simulink model "Arritmia"  (R2023a)
settings: Solver=ode15s  StartTime=0  StopTime=5  MaxStep=1e-3  RelTol=1e-3
libraries: slpidlib x1
settings Model: Creator=piqui  LastModifiedBy=jaelb
settings DataIOCC: ReturnWorkspaceOutputs=off  TimeSaveName=t
settings DebuggingCC: AlgebraicLoopMsg=none  ArtificialAlgebraicLoopMsg=none  MaxConsecutiveZCsMsg=none  ModelReferenceExtraNoncontSigs=none  OperatingPointInterfaceChecksumMismatchMsg=none

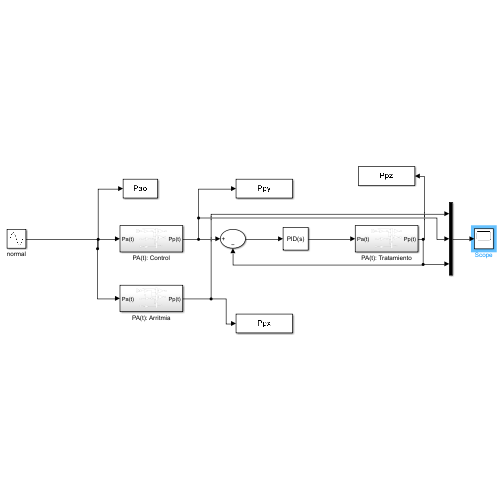
[thumbnail: Simulink's stored preview of the top-level diagram]
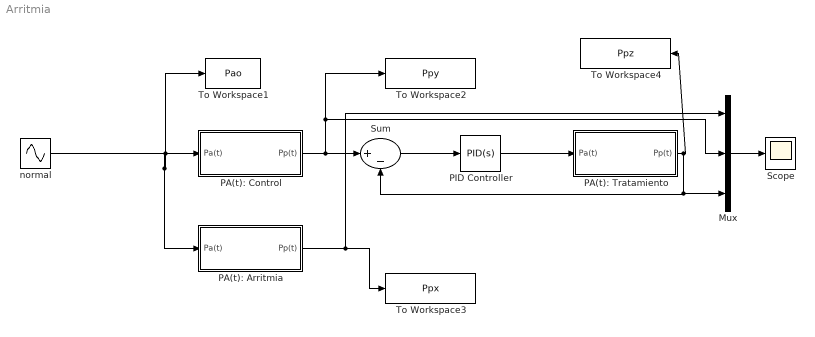
== system Arritmia ==
  Mux : Mux  Inputs=3
  PA(t): Arritmia : Subsystem
  PA(t): Control : Subsystem
  PA(t): Tratamiento : Subsystem
  PID Controller : slpidlib/PID Controller  Controller=PID  Form=Parallel  TimeDomain=Continuous-time  UseExternalTs=off  SampleTime=-1  IntegratorMethod=Forward Euler  FilterMethod=Forward Euler  ControllerParametersSource=internal  P=1382.64108107363  I=23976.1659464632  UseKiTs=off  D=7.06671657792426  N=251170.983745407  UseFilter=on  TunerSelectOption=Transfer Function Based (PID Tuner App)  InitialConditionSource=internal  InitialConditionForIntegrator=0  InitialConditionForFilter=0  DifferentiatorICPrevScaledInput=0  ExternalReset=none  TrackingMode=off  Kt=1  LimitOutput=off  SatLimitsSource=internal  UpperSaturationLimit=inf  LowerSaturationLimit=-inf  LinearizeAsGain=on  AntiWindupMode=none  Kb=1  LimitIntegrator=off  UpperIntegratorSaturationLimit=inf  LowerIntegratorSaturationLimit=-inf  POutMin=[]  POutMax=[]  IOutMin=[]  IOutMax=[]  DOutMin=[]  DOutMax=[]  NOutMin=[]  NOutMax=[]  SumOutMin=[]  SumOutMax=[]  SaturationOutMin=[]  SaturationOutMax=[]  PParamMin=[]  PParamMax=[]  IParamMin=[]  IParamMax=[]  DParamMin=[]  DParamMax=[]  NParamMin=[]  NParamMax=[]  KbParamMin=[]  KbParamMax=[]  KtParamMin=[]  KtParamMax=[]  KbOutMin=[]  KbOutMax=[]  KtOutMin=[]  KtOutMax=[]  IntegratorOutMin=[]  IntegratorOutMax=[]  FilterOutMin=[]  FilterOutMax=[]  SumI1OutMin=[]  SumI1OutMax=[]  SumI2OutMin=[]  SumI2OutMax=[]  SumI3OutMin=[]  SumI3OutMax=[]  SumI4OutMin=[]  SumI4OutMax=[]  SumDOutMin=[]  SumDOutMax=[]  DifferentiatorOutMin=[]  DifferentiatorOutMax=[]  FilterDiffOutCoefMin=[]  FilterDiffOutCoefMax=[]  ReciprocalOutMin=[]  ReciprocalOutMax=[]  SumDenOutMin=[]  SumDenOutMax=[]  SumNumOutMin=[]  SumNumOutMax=[]  DivideOutMin=[]  DivideOutMax=[]  UdiffTsProdOutMin=[]  UdiffTsProdOutMax=[]  NTsProdOutMin=[]  NTsProdOutMax=[]  UintegralTsProdOutMin=[]  UintegralTsProdOutMax=[]  UngainTsProdOutMin=[]  UngainTsProdOutMax=[]  ClampingZeroOutDataTypeStr=Inherit: Inherit via back propagation  ClampingZeroOutMin=[]  ClampingZeroOutMax=[]  FilterDenConstantOutDataTypeStr=Inherit: Inherit via back propagation  FilterDenConstantOutMin=[]  FilterDenConstantOutMax=[]  PCopyOutDataTypeStr=Inherit: Inherit via back propagation  PCopyOutMin=[]  PCopyOutMax=[]  NCopyOutDataTypeStr=Inherit: Inherit via back propagation  NCopyOutMin=[]  NCopyOutMax=[]  IntegratorContinuousStateAttributes=''  IntegratorStateMustResolveToSignalObject=off  IntegratorRTWStateStorageClass=Auto  FilterContinuousStateAttributes=''  FilterStateMustResolveToSignalObject=off  FilterRTWStateStorageClass=Auto  ParallelPVariant=InternalParameters  IdealPVariant=Disabled  IVariant=InternalParameters  DVariant=InternalParameters  IntegratorVariant=Continuous  SatVariant=Disabled  AWVariant=Passthrough  PCopyVariant=Disabled  TRVariant=Disabled  FdbkBlocksVariant=Forward  IdealPFdbkVariant=Disabled  SatFdbkVariant=Disabled  DerivativeFilterVariant=ContFilter  NVariant=InternalParameters  NCopyVariant=Disabled  FilterICVariant=InternalICsFilter  IntegratorICVariant=InternalICs  ExternalResetVariant=Disabled  TRSumVariant=Passthrough  SumFdbkVariant=Disabled  SumVariant=Sum_PID  TsampFilterVariant=InternalTs  TsampNgainVariant=Passthrough  TsampIntegralVariant=Disabled_SignalSpec  ExternalSaturationOutDataTypeStr=Inherit: Same as second input
  Scope : Scope
  Sum : Sum  Inputs=|+-
  To Workspace1 : ToWorkspace  VariableName=Pao  SampleTime=-1
  To Workspace2 : ToWorkspace  VariableName=Ppy  SampleTime=-1
  To Workspace3 : ToWorkspace  VariableName=Ppx  SampleTime=-1
  To Workspace4 : ToWorkspace  VariableName=Ppz  SampleTime=-1
  normal : Sin  Frequency=pi*2  SampleTime=0
  wires:
  normal/1 -> PA(t): Arritmia/1(Pa(t)), PA(t): Control/1(Pa(t)), To Workspace1/1
  Sum/1 -> PID Controller/1
  Mux/1 -> Scope/1
  PA(t): Control/1(Pp(t)) -> Mux/2, To Workspace2/1, Sum/1
  PA(t): Arritmia/1(Pp(t)) -> Mux/1, To Workspace3/1
  PID Controller/1 -> PA(t): Tratamiento/1(Pa(t))
  PA(t): Tratamiento/1(Pp(t)) -> Mux/3, Sum/2, To Workspace4/1

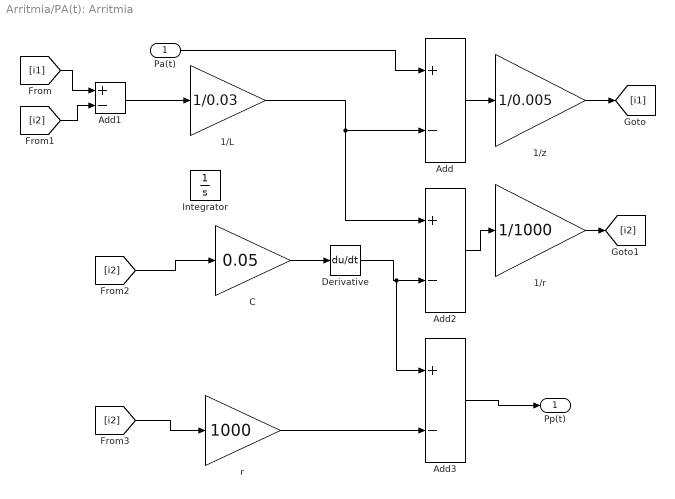
== system Arritmia/PA(t): Arritmia ==
  Pa(t) : Inport
  1/L : Gain  Gain=1/0.03
  1/r : Gain  Gain=1/1000
  1/z : Gain  Gain=1/0.005
  Add{,1..3} (4 alike) : Sum  Inputs=+-
  C : Gain  Gain=0.05
  Derivative : Derivative
  Integrator : Integrator
  r : Gain  Gain=1000
  Pp(t) : Outport
  wires:
  1/L/1 -> Add2/1, Add/2
  1/z/1 -> [i1]
  [i1] -> Add1/1
  Add2/1 -> 1/r/1
  Add3/1 -> Pp(t)/1
  r/1 -> Add3/2
  Pa(t)/1 -> Add/1
  Add/1 -> 1/z/1
  Derivative/1 -> Add3/1, Add2/2
  Add1/1 -> 1/L/1
  1/r/1 -> [i2]
  C/1 -> Derivative/1
  [i2] -> Add1/2
  [i2] -> C/1
  [i2] -> r/1

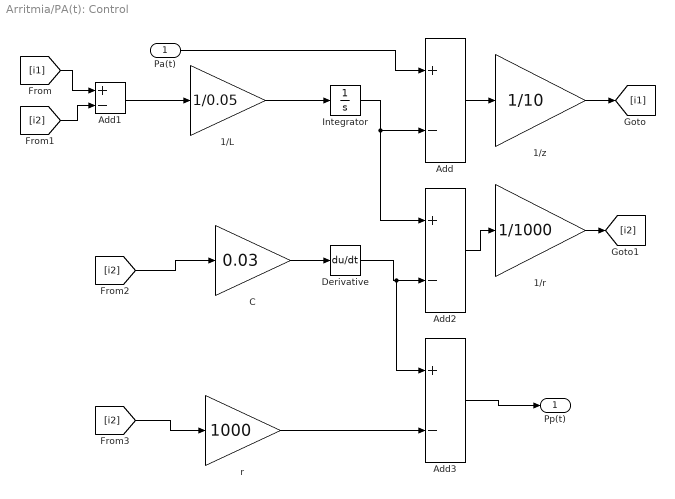
== system Arritmia/PA(t): Control ==
  Pa(t) : Inport
  1/L : Gain  Gain=1/0.05
  1/r : Gain  Gain=1/1000
  1/z : Gain  Gain=1/10
  Add{,1..3} (4 alike) : Sum  Inputs=+-
  C : Gain  Gain=0.03
  Derivative : Derivative
  Integrator : Integrator
  r : Gain  Gain=1000
  Pp(t) : Outport
  wires:
  Add3/1 -> Pp(t)/1
  r/1 -> Add3/2
  Add1/1 -> 1/L/1
  [i2] -> r/1
  1/r/1 -> [i2]
  Integrator/1 -> Add2/1, Add/2
  Derivative/1 -> Add3/1, Add2/2
  [i2] -> Add1/2
  [i2] -> C/1
  Pa(t)/1 -> Add/1
  [i1] -> Add1/1
  Add2/1 -> 1/r/1
  1/z/1 -> [i1]
  Add/1 -> 1/z/1
  1/L/1 -> Integrator/1
  C/1 -> Derivative/1

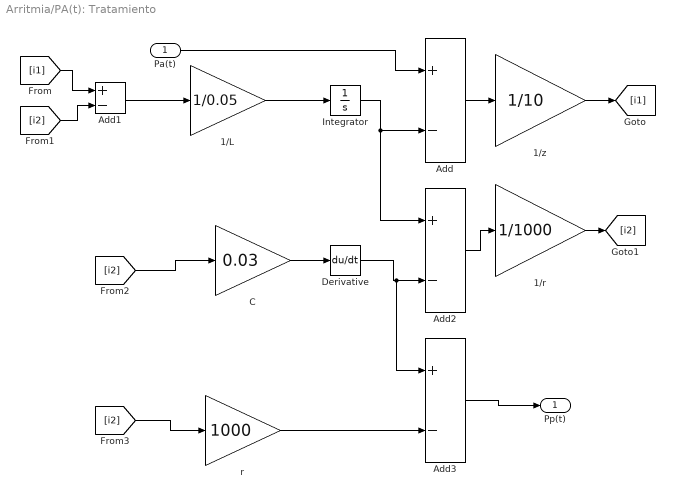
== system Arritmia/PA(t): Tratamiento ==
  Pa(t) : Inport
  1/L : Gain  Gain=1/0.05
  1/r : Gain  Gain=1/1000
  1/z : Gain  Gain=1/10
  Add{,1..3} (4 alike) : Sum  Inputs=+-
  C : Gain  Gain=0.03
  Derivative : Derivative
  Integrator : Integrator
  r : Gain  Gain=1000
  Pp(t) : Outport
  wires:
  Add3/1 -> Pp(t)/1
  r/1 -> Add3/2
  Add1/1 -> 1/L/1
  [i2] -> r/1
  1/r/1 -> [i2]
  Integrator/1 -> Add2/1, Add/2
  Derivative/1 -> Add3/1, Add2/2
  [i2] -> Add1/2
  [i2] -> C/1
  Pa(t)/1 -> Add/1
  [i1] -> Add1/1
  Add2/1 -> 1/r/1
  1/z/1 -> [i1]
  Add/1 -> 1/z/1
  1/L/1 -> Integrator/1
  C/1 -> Derivative/1
